simulink model "gm_sampleModel71194_pp_7_1_sub"  (R2023b)
settings: Solver=VariableStepAuto  StartTime=0.0  StopTime=10.0  RelTol=1e-3
libraries: simulink x45, hdlsllib x1, hdlmdlgenlib x1
(part 2 of 2)

== system gm_sampleModel71194_pp_7_1_sub/Subsystem/cfblk214 ==
  emi_180 : Inport  OutDataTypeStr=boolean  PortDimensions=1  SampleTime=1
  Action Port : Inport  Port=2  OutDataTypeStr=boolean  SampleTime=1
  cfblk214 : DataTypeConversion  OutDataTypeStr=uint8  SampleTime=1  SaturateOnIntegerOverflow=off  RndMeth=Floor
  cfblk214_out1bypassMux : MultiPortSwitch  DataPortOrder=Zero-based contiguous  Inputs=2  zeroidx=on  OutDataTypeStr=uint8  SampleTime=1  SaturateOnIntegerOverflow=off  InputSameDT=off
  emi_181_bypass : UnitDelay  InitialCondition="fi(0,0,8,0,\"hex\",\"00\")"  SampleTime=1
  emi_181 : Outport  SampleTime=1  InitialOutput=0
  wires:
  Action Port/1 -> cfblk214_out1bypassMux/1
  emi_180/1 -> cfblk214/1
  cfblk214/1 -> cfblk214_out1bypassMux/3
  cfblk214_out1bypassMux/1 -> emi_181_bypass/1, emi_181/1
  emi_181_bypass/1 -> cfblk214_out1bypassMux/2

== system gm_sampleModel71194_pp_7_1_sub/Subsystem/cfblk216 ==
  emi_188 : Inport  OutDataTypeStr=uint8  PortDimensions=1  SampleTime=1
  Action Port : Inport  Port=2  OutDataTypeStr=boolean  SampleTime=1
  cfblk216 : DataTypeConversion  OutDataTypeStr=fixdt(0,8,0)
  cfblk216_out1bypassMux : MultiPortSwitch  DataPortOrder=Zero-based contiguous  Inputs=2  zeroidx=on  OutDataTypeStr=uint8  SampleTime=1  SaturateOnIntegerOverflow=off  InputSameDT=off
  emi_189_bypass : UnitDelay  InitialCondition="fi(0,0,8,0,\"hex\",\"00\")"  SampleTime=1
  emi_189 : Outport  SampleTime=1  InitialOutput=0
  wires:
  Action Port/1 -> cfblk216_out1bypassMux/1
  emi_188/1 -> cfblk216/1
  cfblk216/1 -> cfblk216_out1bypassMux/3
  cfblk216_out1bypassMux/1 -> emi_189_bypass/1, emi_189/1
  emi_189_bypass/1 -> cfblk216_out1bypassMux/2

== system gm_sampleModel71194_pp_7_1_sub/Subsystem/cfblk217 ==
  emi_196 : Inport  OutDataTypeStr=fixdt(0, 16, 7)  PortDimensions=1  SampleTime=1
  Action Port : Inport  Port=2  OutDataTypeStr=boolean  SampleTime=1
  cfblk217 : DataTypeConversion  OutDataTypeStr=uint8  SampleTime=1  SaturateOnIntegerOverflow=off  RndMeth=Floor
  cfblk217_out1bypassMux : MultiPortSwitch  DataPortOrder=Zero-based contiguous  Inputs=2  zeroidx=on  OutDataTypeStr=uint8  SampleTime=1  SaturateOnIntegerOverflow=off  InputSameDT=off
  emi_197_bypass : UnitDelay  InitialCondition="fi(0,0,8,0,\"hex\",\"00\")"  SampleTime=1
  emi_197 : Outport  SampleTime=1  InitialOutput=0
  wires:
  Action Port/1 -> cfblk217_out1bypassMux/1
  emi_196/1 -> cfblk217/1
  cfblk217/1 -> cfblk217_out1bypassMux/3
  cfblk217_out1bypassMux/1 -> emi_197_bypass/1, emi_197/1
  emi_197_bypass/1 -> cfblk217_out1bypassMux/2

== system gm_sampleModel71194_pp_7_1_sub/Subsystem/cfblk220 ==
  emi_230 : Inport  OutDataTypeStr=uint8  PortDimensions=1  SampleTime=1
  Action Port : Inport  Port=2  OutDataTypeStr=boolean  SampleTime=1
  cfblk220 : DataTypeConversion  OutDataTypeStr=fixdt(0,8,0)
  cfblk220_out1bypassMux : MultiPortSwitch  DataPortOrder=Zero-based contiguous  Inputs=2  zeroidx=on  OutDataTypeStr=uint8  SampleTime=1  SaturateOnIntegerOverflow=off  InputSameDT=off
  emi_231_bypass : UnitDelay  InitialCondition="fi(0,0,8,0,\"hex\",\"00\")"  SampleTime=1
  emi_231 : Outport  SampleTime=1  InitialOutput=0
  wires:
  Action Port/1 -> cfblk220_out1bypassMux/1
  emi_230/1 -> cfblk220/1
  cfblk220/1 -> cfblk220_out1bypassMux/3
  cfblk220_out1bypassMux/1 -> emi_231_bypass/1, emi_231/1
  emi_231_bypass/1 -> cfblk220_out1bypassMux/2

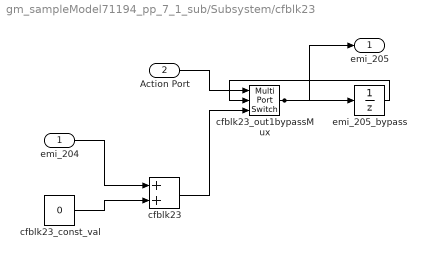
== system gm_sampleModel71194_pp_7_1_sub/Subsystem/cfblk23 ==
  emi_204 : Inport  OutDataTypeStr=uint8  PortDimensions=1  SampleTime=1
  Action Port : Inport  Port=2  OutDataTypeStr=boolean  SampleTime=1
  cfblk23 : Sum  OutDataTypeStr=uint8  AccumDataTypeStr=uint8  RndMeth=Nearest  SampleTime=1
  cfblk23_const_val : Constant  Value=0  VectorParams1D=off  OutDataTypeStr=uint8  SampleTime=1
  cfblk23_out1bypassMux : MultiPortSwitch  DataPortOrder=Zero-based contiguous  Inputs=2  zeroidx=on  OutDataTypeStr=uint8  SampleTime=1  SaturateOnIntegerOverflow=off  InputSameDT=off
  emi_205_bypass : UnitDelay  InitialCondition="fi(0,0,8,0,\"hex\",\"00\")"  SampleTime=1
  emi_205 : Outport  SampleTime=1  InitialOutput=0
  wires:
  Action Port/1 -> cfblk23_out1bypassMux/1
  emi_204/1 -> cfblk23/1
  cfblk23/1 -> cfblk23_out1bypassMux/3
  cfblk23_out1bypassMux/1 -> emi_205_bypass/1, emi_205/1
  emi_205_bypass/1 -> cfblk23_out1bypassMux/2
  cfblk23_const_val/1 -> cfblk23/2

== system gm_sampleModel71194_pp_7_1_sub/Subsystem/cfblk27 ==
  emi_164 : Inport  OutDataTypeStr=uint8  PortDimensions=1  SampleTime=1
  Action Port : Inport  Port=2  OutDataTypeStr=boolean  SampleTime=1
  cfblk27 : Abs  SampleTime=1  OutDataTypeStr=uint8  SaturateOnIntegerOverflow=off
  cfblk27_out1bypassMux : MultiPortSwitch  DataPortOrder=Zero-based contiguous  Inputs=2  zeroidx=on  OutDataTypeStr=uint8  SampleTime=1  SaturateOnIntegerOverflow=off  InputSameDT=off
  emi_165_bypass : UnitDelay  InitialCondition="fi(0,0,8,0,\"hex\",\"00\")"  SampleTime=1
  emi_165 : Outport  SampleTime=1  InitialOutput=0
  wires:
  Action Port/1 -> cfblk27_out1bypassMux/1
  emi_164/1 -> cfblk27/1
  cfblk27/1 -> cfblk27_out1bypassMux/3
  cfblk27_out1bypassMux/1 -> emi_165_bypass/1, emi_165/1
  emi_165_bypass/1 -> cfblk27_out1bypassMux/2

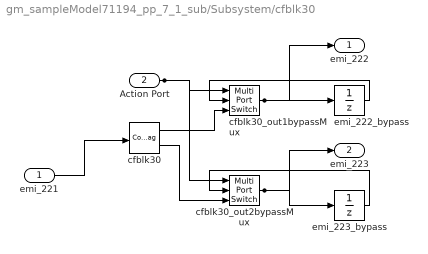
== system gm_sampleModel71194_pp_7_1_sub/Subsystem/cfblk30 ==
  emi_221 : Inport  OutDataTypeStr=uint8  PortDimensions=1  SampleTime=1
  Action Port : Inport  Port=2  OutDataTypeStr=boolean  SampleTime=1
  cfblk30 : ComplexToRealImag  SampleTime=1
  cfblk30_out1bypassMux : MultiPortSwitch  DataPortOrder=Zero-based contiguous  Inputs=2  zeroidx=on  OutDataTypeStr=uint8  SampleTime=1  SaturateOnIntegerOverflow=off  InputSameDT=off
  cfblk30_out2bypassMux : MultiPortSwitch  DataPortOrder=Zero-based contiguous  Inputs=2  zeroidx=on  OutDataTypeStr=uint8  SampleTime=1  SaturateOnIntegerOverflow=off  InputSameDT=off
  emi_222_bypass : UnitDelay  InitialCondition="fi(0,0,8,0,\"hex\",\"00\")"  SampleTime=1
  emi_223_bypass : UnitDelay  InitialCondition="fi(0,0,8,0,\"hex\",\"00\")"  SampleTime=1
  emi_222 : Outport  SampleTime=1  InitialOutput=0
  emi_223 : Outport  Port=2  SampleTime=1  InitialOutput=0
  wires:
  Action Port/1 -> cfblk30_out2bypassMux/1, cfblk30_out1bypassMux/1
  emi_221/1 -> cfblk30/1
  cfblk30/1 -> cfblk30_out1bypassMux/3
  cfblk30/2 -> cfblk30_out2bypassMux/3
  cfblk30_out1bypassMux/1 -> emi_222_bypass/1, emi_222/1
  emi_222_bypass/1 -> cfblk30_out1bypassMux/2
  cfblk30_out2bypassMux/1 -> emi_223_bypass/1, emi_223/1
  emi_223_bypass/1 -> cfblk30_out2bypassMux/2

== system gm_sampleModel71194_pp_7_1_sub/Subsystem/cfblk31_inst ==
  in1 : Inport  OutDataTypeStr=uint8  SampleTime=1
  in2 : Inport  Port=2  OutDataTypeStr=uint8  SampleTime=1
  mul_cfblk31_dotp_mulcomp : Product  Inputs=**  OutDataTypeStr=uint8  SampleTime=1
  out1 : Outport  OutDataTypeStr=uint8  SampleTime=1
  wires:
  in1/1 -> mul_cfblk31_dotp_mulcomp/1
  in2/1 -> mul_cfblk31_dotp_mulcomp/2
  mul_cfblk31_dotp_mulcomp/1 -> out1/1

== system gm_sampleModel71194_pp_7_1_sub/Subsystem/cfblk37 ==
  emi_238 : Inport  OutDataTypeStr=uint8  PortDimensions=1  SampleTime=1
  Action Port : Inport  Port=2  OutDataTypeStr=boolean  SampleTime=1
  cfblk37 : MinMax
  cfblk37_out1bypassMux : MultiPortSwitch  DataPortOrder=Zero-based contiguous  Inputs=2  zeroidx=on  OutDataTypeStr=uint8  SampleTime=1  SaturateOnIntegerOverflow=off  InputSameDT=off
  emi_239_bypass : UnitDelay  InitialCondition="fi(0,0,8,0,\"hex\",\"00\")"  SampleTime=1
  emi_239 : Outport  SampleTime=1  InitialOutput=0
  wires:
  Action Port/1 -> cfblk37_out1bypassMux/1
  emi_238/1 -> cfblk37/1
  cfblk37/1 -> cfblk37_out1bypassMux/3
  cfblk37_out1bypassMux/1 -> emi_239_bypass/1, emi_239/1
  emi_239_bypass/1 -> cfblk37_out1bypassMux/2

== system gm_sampleModel71194_pp_7_1_sub/Subsystem/cfblk38 ==
  u : Inport  OutDataTypeStr=uint8  SampleTime=1
  FixPt Constant : Constant  DisableCoverage=on  OutDataTypeStr=Inherit: Inherit via back propagation  SampleTime=-1
  FixPt Data Type Duplicate : DataTypeDuplicate  DisableCoverage=on  NumInputPorts=3
  FixPt Sum1 : Sum  OutDataTypeStr=Inherit: Inherit via back propagation  InputSameDT=on  LockScale=on
  y : Outport  SampleTime=1
  wires:
  u/1 -> FixPt Sum1/1, FixPt Data Type Duplicate/2
  FixPt Constant/1 -> FixPt Sum1/2, FixPt Data Type Duplicate/3
  FixPt Sum1/1 -> FixPt Data Type Duplicate/1, y/1

== system gm_sampleModel71194_pp_7_1_sub/Subsystem/cfblk39 ==
  emi_246 : Inport  OutDataTypeStr=uint8  PortDimensions=1  SampleTime=1
  Action Port : Inport  Port=2  OutDataTypeStr=boolean  SampleTime=1
  cfblk39 : Subsystem  mask(Real World Value Increment){}
      mask help: Simulink:masks:RealWorldValueIncrement_MD
      mask Display: disp('V++')
  cfblk39_out1bypassMux : MultiPortSwitch  DataPortOrder=Zero-based contiguous  Inputs=2  zeroidx=on  OutDataTypeStr=uint8  SampleTime=1  SaturateOnIntegerOverflow=off  InputSameDT=off
  emi_247_bypass : UnitDelay  InitialCondition="fi(0,0,8,0,\"hex\",\"00\")"  SampleTime=1
  emi_247 : Outport  SampleTime=1  InitialOutput=0
  wires:
  Action Port/1 -> cfblk39_out1bypassMux/1
  emi_246/1 -> cfblk39/1(u)
  cfblk39/1(y) -> cfblk39_out1bypassMux/3
  cfblk39_out1bypassMux/1 -> emi_247_bypass/1, emi_247/1
  emi_247_bypass/1 -> cfblk39_out1bypassMux/2

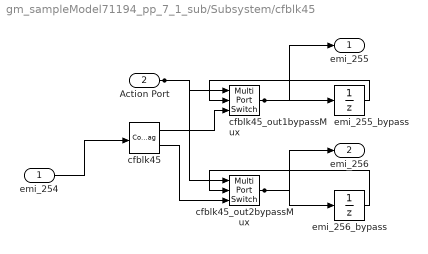
== system gm_sampleModel71194_pp_7_1_sub/Subsystem/cfblk45 ==
  emi_254 : Inport  OutDataTypeStr=uint8  PortDimensions=1  SampleTime=1
  Action Port : Inport  Port=2  OutDataTypeStr=boolean  SampleTime=1
  cfblk45 : ComplexToRealImag  SampleTime=1
  cfblk45_out1bypassMux : MultiPortSwitch  DataPortOrder=Zero-based contiguous  Inputs=2  zeroidx=on  OutDataTypeStr=uint8  SampleTime=1  SaturateOnIntegerOverflow=off  InputSameDT=off
  cfblk45_out2bypassMux : MultiPortSwitch  DataPortOrder=Zero-based contiguous  Inputs=2  zeroidx=on  OutDataTypeStr=uint8  SampleTime=1  SaturateOnIntegerOverflow=off  InputSameDT=off
  emi_255_bypass : UnitDelay  InitialCondition="fi(0,0,8,0,\"hex\",\"00\")"  SampleTime=1
  emi_256_bypass : UnitDelay  InitialCondition="fi(0,0,8,0,\"hex\",\"00\")"  SampleTime=1
  emi_255 : Outport  SampleTime=1  InitialOutput=0
  emi_256 : Outport  Port=2  SampleTime=1  InitialOutput=0
  wires:
  Action Port/1 -> cfblk45_out2bypassMux/1, cfblk45_out1bypassMux/1
  emi_254/1 -> cfblk45/1
  cfblk45/1 -> cfblk45_out1bypassMux/3
  cfblk45/2 -> cfblk45_out2bypassMux/3
  cfblk45_out1bypassMux/1 -> emi_255_bypass/1, emi_255/1
  emi_255_bypass/1 -> cfblk45_out1bypassMux/2
  cfblk45_out2bypassMux/1 -> emi_256_bypass/1, emi_256/1
  emi_256_bypass/1 -> cfblk45_out2bypassMux/2

== system gm_sampleModel71194_pp_7_1_sub/Subsystem/cfblk46 ==
  emi_263 : Inport  OutDataTypeStr=uint8  PortDimensions=1  SampleTime=1
  Action Port : Inport  Port=2  OutDataTypeStr=boolean  SampleTime=1
  cfblk46 : Sum  Inputs=+
  cfblk46_out1bypassMux : MultiPortSwitch  DataPortOrder=Zero-based contiguous  Inputs=2  zeroidx=on  OutDataTypeStr=uint8  SampleTime=1  SaturateOnIntegerOverflow=off  InputSameDT=off
  emi_264_bypass : UnitDelay  InitialCondition="fi(0,0,8,0,\"hex\",\"00\")"  SampleTime=1
  emi_264 : Outport  SampleTime=1  InitialOutput=0
  wires:
  Action Port/1 -> cfblk46_out1bypassMux/1
  emi_263/1 -> cfblk46/1
  cfblk46/1 -> cfblk46_out1bypassMux/3
  cfblk46_out1bypassMux/1 -> emi_264_bypass/1, emi_264/1
  emi_264_bypass/1 -> cfblk46_out1bypassMux/2

== system gm_sampleModel71194_pp_7_1_sub/Subsystem/cfblk50 ==
  emi_271 : Inport  OutDataTypeStr=uint8  PortDimensions=1  SampleTime=1
  Action Port : Inport  Port=2  OutDataTypeStr=boolean  SampleTime=1
  cfblk50 : Sum  Inputs=+
  cfblk50_out1bypassMux : MultiPortSwitch  DataPortOrder=Zero-based contiguous  Inputs=2  zeroidx=on  OutDataTypeStr=uint8  SampleTime=1  SaturateOnIntegerOverflow=off  InputSameDT=off
  emi_272_bypass : UnitDelay  InitialCondition="fi(0,0,8,0,\"hex\",\"00\")"  SampleTime=1
  emi_272 : Outport  SampleTime=1  InitialOutput=0
  wires:
  Action Port/1 -> cfblk50_out1bypassMux/1
  emi_271/1 -> cfblk50/1
  cfblk50/1 -> cfblk50_out1bypassMux/3
  cfblk50_out1bypassMux/1 -> emi_272_bypass/1, emi_272/1
  emi_272_bypass/1 -> cfblk50_out1bypassMux/2

== system gm_sampleModel71194_pp_7_1_sub/Subsystem/cfblk52 ==
  u : Inport  OutDataTypeStr=uint8  SampleTime=1
  FixPt Constant : Constant  DisableCoverage=on  OutDataTypeStr=Inherit: Inherit via back propagation  SampleTime=-1
  FixPt Data Type Duplicate : DataTypeDuplicate  DisableCoverage=on  NumInputPorts=3
  FixPt Sum1 : Sum  OutDataTypeStr=Inherit: Inherit via back propagation  InputSameDT=on  LockScale=on
  y : Outport  SampleTime=1
  wires:
  u/1 -> FixPt Sum1/1, FixPt Data Type Duplicate/2
  FixPt Constant/1 -> FixPt Sum1/2, FixPt Data Type Duplicate/3
  FixPt Sum1/1 -> FixPt Data Type Duplicate/1, y/1

== system gm_sampleModel71194_pp_7_1_sub/Subsystem/cfblk54 ==
  emi_279 : Inport  OutDataTypeStr=uint8  PortDimensions=1  SampleTime=1
  Action Port : Inport  Port=2  OutDataTypeStr=boolean  SampleTime=1
  cfblk54 : MinMax
  cfblk54_out1bypassMux : MultiPortSwitch  DataPortOrder=Zero-based contiguous  Inputs=2  zeroidx=on  OutDataTypeStr=uint8  SampleTime=1  SaturateOnIntegerOverflow=off  InputSameDT=off
  emi_280_bypass : UnitDelay  InitialCondition="fi(0,0,8,0,\"hex\",\"00\")"  SampleTime=1
  emi_280 : Outport  SampleTime=1  InitialOutput=0
  wires:
  Action Port/1 -> cfblk54_out1bypassMux/1
  emi_279/1 -> cfblk54/1
  cfblk54/1 -> cfblk54_out1bypassMux/3
  cfblk54_out1bypassMux/1 -> emi_280_bypass/1, emi_280/1
  emi_280_bypass/1 -> cfblk54_out1bypassMux/2

== system gm_sampleModel71194_pp_7_1_sub/Subsystem/cfblk55 ==
  u : Inport  OutDataTypeStr=uint8  SampleTime=1
  FixPt Constant : Constant  DisableCoverage=on  OutDataTypeStr=Inherit: Inherit via back propagation  SampleTime=-1
  FixPt Data Type Duplicate : DataTypeDuplicate  DisableCoverage=on  NumInputPorts=3
  FixPt Sum1 : Sum  OutDataTypeStr=Inherit: Inherit via back propagation  InputSameDT=on  LockScale=on
  y : Outport  SampleTime=1
  wires:
  u/1 -> FixPt Sum1/1, FixPt Data Type Duplicate/2
  FixPt Constant/1 -> FixPt Sum1/2, FixPt Data Type Duplicate/3
  FixPt Sum1/1 -> FixPt Data Type Duplicate/1, y/1

== system gm_sampleModel71194_pp_7_1_sub/Subsystem/cfblk6 ==
  emi_287 : Inport  OutDataTypeStr=boolean  PortDimensions=1  SampleTime=1
  Action Port : Inport  Port=2  OutDataTypeStr=boolean  SampleTime=1
  cfblk6 : simulink/Logic and Bit Operations/Bitwise Operator  logicop=AND  UseBitMask=on  BitMask="fi(0,0,1,0,\"hex\",\"1\")"  BitMaskRealWorld=Real World Value
  cfblk6_out1bypassMux : MultiPortSwitch  DataPortOrder=Zero-based contiguous  Inputs=2  zeroidx=on  SampleTime=1  SaturateOnIntegerOverflow=off  InputSameDT=off
  emi_288_bypass : UnitDelay  SampleTime=1
  emi_288 : Outport  SampleTime=1  InitialOutput=0
  wires:
  Action Port/1 -> cfblk6_out1bypassMux/1
  emi_287/1 -> cfblk6/1
  cfblk6/1 -> cfblk6_out1bypassMux/3
  cfblk6_out1bypassMux/1 -> emi_288_bypass/1, emi_288/1
  emi_288_bypass/1 -> cfblk6_out1bypassMux/2

== system gm_sampleModel71194_pp_7_1_sub/Subsystem/cfblk60 ==
  u : Inport  OutDataTypeStr=uint8  SampleTime=1
  FixPt Constant : Constant  DisableCoverage=on  OutDataTypeStr=Inherit: Inherit via back propagation  SampleTime=-1
  FixPt Data Type Duplicate : DataTypeDuplicate  DisableCoverage=on  NumInputPorts=3
  FixPt Sum1 : Sum  OutDataTypeStr=Inherit: Inherit via back propagation  InputSameDT=on  LockScale=on
  y : Outport  SampleTime=1
  wires:
  u/1 -> FixPt Sum1/1, FixPt Data Type Duplicate/2
  FixPt Constant/1 -> FixPt Sum1/2, FixPt Data Type Duplicate/3
  FixPt Sum1/1 -> FixPt Data Type Duplicate/1, y/1

== system gm_sampleModel71194_pp_7_1_sub/Subsystem/cfblk63 ==
  emi_295 : Inport  OutDataTypeStr=uint8  PortDimensions=1  SampleTime=1
  Action Port : Inport  Port=2  OutDataTypeStr=boolean  SampleTime=1
  cfblk63 : Subsystem  mask(Real World Value Increment){}
      mask help: Simulink:masks:RealWorldValueIncrement_MD
      mask Display: disp('V++')
  cfblk63_out1bypassMux : MultiPortSwitch  DataPortOrder=Zero-based contiguous  Inputs=2  zeroidx=on  OutDataTypeStr=uint8  SampleTime=1  SaturateOnIntegerOverflow=off  InputSameDT=off
  emi_296_bypass : UnitDelay  InitialCondition="fi(0,0,8,0,\"hex\",\"00\")"  SampleTime=1
  emi_296 : Outport  SampleTime=1  InitialOutput=0
  wires:
  Action Port/1 -> cfblk63_out1bypassMux/1
  emi_295/1 -> cfblk63/1(u)
  cfblk63/1(y) -> cfblk63_out1bypassMux/3
  cfblk63_out1bypassMux/1 -> emi_296_bypass/1, emi_296/1
  emi_296_bypass/1 -> cfblk63_out1bypassMux/2

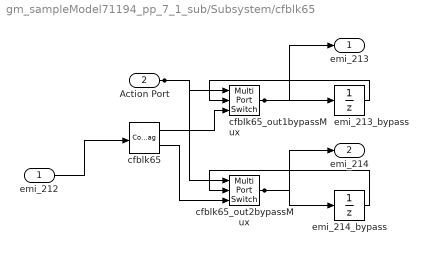
== system gm_sampleModel71194_pp_7_1_sub/Subsystem/cfblk65 ==
  emi_212 : Inport  OutDataTypeStr=uint8  PortDimensions=1  SampleTime=1
  Action Port : Inport  Port=2  OutDataTypeStr=boolean  SampleTime=1
  cfblk65 : ComplexToRealImag  SampleTime=1
  cfblk65_out1bypassMux : MultiPortSwitch  DataPortOrder=Zero-based contiguous  Inputs=2  zeroidx=on  OutDataTypeStr=uint8  SampleTime=1  SaturateOnIntegerOverflow=off  InputSameDT=off
  cfblk65_out2bypassMux : MultiPortSwitch  DataPortOrder=Zero-based contiguous  Inputs=2  zeroidx=on  OutDataTypeStr=uint8  SampleTime=1  SaturateOnIntegerOverflow=off  InputSameDT=off
  emi_213_bypass : UnitDelay  InitialCondition="fi(0,0,8,0,\"hex\",\"00\")"  SampleTime=1
  emi_214_bypass : UnitDelay  InitialCondition="fi(0,0,8,0,\"hex\",\"00\")"  SampleTime=1
  emi_213 : Outport  SampleTime=1  InitialOutput=0
  emi_214 : Outport  Port=2  SampleTime=1  InitialOutput=0
  wires:
  Action Port/1 -> cfblk65_out2bypassMux/1, cfblk65_out1bypassMux/1
  emi_212/1 -> cfblk65/1
  cfblk65/1 -> cfblk65_out1bypassMux/3
  cfblk65/2 -> cfblk65_out2bypassMux/3
  cfblk65_out1bypassMux/1 -> emi_213_bypass/1, emi_213/1
  emi_213_bypass/1 -> cfblk65_out1bypassMux/2
  cfblk65_out2bypassMux/1 -> emi_214_bypass/1, emi_214/1
  emi_214_bypass/1 -> cfblk65_out2bypassMux/2

== system gm_sampleModel71194_pp_7_1_sub/Subsystem/cfblk67 ==
  emi_303 : Inport  OutDataTypeStr=uint8  PortDimensions=1  SampleTime=1
  Action Port : Inport  Port=2  OutDataTypeStr=boolean  SampleTime=1
  cfblk67 : Subsystem  mask(Real World Value Increment){}
      mask help: Simulink:masks:RealWorldValueIncrement_MD
      mask Display: disp('V++')
  cfblk67_out1bypassMux : MultiPortSwitch  DataPortOrder=Zero-based contiguous  Inputs=2  zeroidx=on  OutDataTypeStr=uint8  SampleTime=1  SaturateOnIntegerOverflow=off  InputSameDT=off
  emi_304_bypass : UnitDelay  InitialCondition="fi(0,0,8,0,\"hex\",\"00\")"  SampleTime=1
  emi_304 : Outport  SampleTime=1  InitialOutput=0
  wires:
  Action Port/1 -> cfblk67_out1bypassMux/1
  emi_303/1 -> cfblk67/1(u)
  cfblk67/1(y) -> cfblk67_out1bypassMux/3
  cfblk67_out1bypassMux/1 -> emi_304_bypass/1, emi_304/1
  emi_304_bypass/1 -> cfblk67_out1bypassMux/2

== system gm_sampleModel71194_pp_7_1_sub/Subsystem/cfblk7 ==
  u : Inport  OutDataTypeStr=uint8  SampleTime=1
  Compare : RelationalOperator  Operator=<=  OutDataTypeStr=fixdt(0, 8)
  Constant : Constant  DisableCoverage=on  Value=0  OutDataTypeStr=Inherit: Inherit via back propagation  SampleTime=-1  PreserveConstantTs=on
  y : Outport  SampleTime=1
  wires:
  u/1 -> Compare/1
  Compare/1 -> y/1
  Constant/1 -> Compare/2

== system gm_sampleModel71194_pp_7_1_sub/Subsystem/cfblk75 ==
  u : Inport  OutDataTypeStr=uint8  SampleTime=1
  FixPt Constant : Constant  DisableCoverage=on  OutDataTypeStr=Inherit: Inherit via back propagation  SampleTime=-1
  FixPt Data Type Duplicate : DataTypeDuplicate  DisableCoverage=on  NumInputPorts=3
  FixPt Sum1 : Sum  OutDataTypeStr=Inherit: Inherit via back propagation  InputSameDT=on  LockScale=on
  y : Outport  SampleTime=1
  wires:
  u/1 -> FixPt Sum1/1, FixPt Data Type Duplicate/2
  FixPt Constant/1 -> FixPt Sum1/2, FixPt Data Type Duplicate/3
  FixPt Sum1/1 -> FixPt Data Type Duplicate/1, y/1

== system gm_sampleModel71194_pp_7_1_sub/Subsystem/cfblk87_inst ==
  in1 : Inport  OutDataTypeStr=uint8  SampleTime=1
  in2 : Inport  Port=2  OutDataTypeStr=uint8  SampleTime=1
  mul_cfblk87_dotp_mulcomp : Product  Inputs=**  OutDataTypeStr=uint8  SampleTime=1
  out1 : Outport  OutDataTypeStr=uint8  SampleTime=1
  wires:
  in1/1 -> mul_cfblk87_dotp_mulcomp/1
  in2/1 -> mul_cfblk87_dotp_mulcomp/2
  mul_cfblk87_dotp_mulcomp/1 -> out1/1

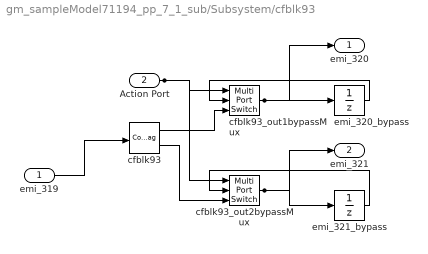
== system gm_sampleModel71194_pp_7_1_sub/Subsystem/cfblk93 ==
  emi_319 : Inport  OutDataTypeStr=uint8  PortDimensions=1  SampleTime=1
  Action Port : Inport  Port=2  OutDataTypeStr=boolean  SampleTime=1
  cfblk93 : ComplexToRealImag  SampleTime=1
  cfblk93_out1bypassMux : MultiPortSwitch  DataPortOrder=Zero-based contiguous  Inputs=2  zeroidx=on  OutDataTypeStr=uint8  SampleTime=1  SaturateOnIntegerOverflow=off  InputSameDT=off
  cfblk93_out2bypassMux : MultiPortSwitch  DataPortOrder=Zero-based contiguous  Inputs=2  zeroidx=on  OutDataTypeStr=uint8  SampleTime=1  SaturateOnIntegerOverflow=off  InputSameDT=off
  emi_320_bypass : UnitDelay  InitialCondition="fi(0,0,8,0,\"hex\",\"00\")"  SampleTime=1
  emi_321_bypass : UnitDelay  InitialCondition="fi(0,0,8,0,\"hex\",\"00\")"  SampleTime=1
  emi_320 : Outport  SampleTime=1  InitialOutput=0
  emi_321 : Outport  Port=2  SampleTime=1  InitialOutput=0
  wires:
  Action Port/1 -> cfblk93_out2bypassMux/1, cfblk93_out1bypassMux/1
  emi_319/1 -> cfblk93/1
  cfblk93/1 -> cfblk93_out1bypassMux/3
  cfblk93/2 -> cfblk93_out2bypassMux/3
  cfblk93_out1bypassMux/1 -> emi_320_bypass/1, emi_320/1
  emi_320_bypass/1 -> cfblk93_out1bypassMux/2
  cfblk93_out2bypassMux/1 -> emi_321_bypass/1, emi_321/1
  emi_321_bypass/1 -> cfblk93_out2bypassMux/2

== system gm_sampleModel71194_pp_7_1_sub/Subsystem/cfblk95 ==
  emi_311 : Inport  OutDataTypeStr=uint8  PortDimensions=1  SampleTime=1
  Action Port : Inport  Port=2  OutDataTypeStr=boolean  SampleTime=1
  cfblk95 : Signum  SampleTime=1
  cfblk95_out1bypassMux : MultiPortSwitch  DataPortOrder=Zero-based contiguous  Inputs=2  zeroidx=on  OutDataTypeStr=uint8  SampleTime=1  SaturateOnIntegerOverflow=off  InputSameDT=off
  emi_312_bypass : UnitDelay  InitialCondition="fi(0,0,8,0,\"hex\",\"00\")"  SampleTime=1
  emi_312 : Outport  SampleTime=1  InitialOutput=0
  wires:
  Action Port/1 -> cfblk95_out1bypassMux/1
  emi_311/1 -> cfblk95/1
  cfblk95/1 -> cfblk95_out1bypassMux/3
  cfblk95_out1bypassMux/1 -> emi_312_bypass/1, emi_312/1
  emi_312_bypass/1 -> cfblk95_out1bypassMux/2

== system gm_sampleModel71194_pp_7_1_sub/Subsystem/cfblk103/cfblk103 ==
  u : Inport  OutDataTypeStr=uint8  SampleTime=1
  FixPt Constant : Constant  DisableCoverage=on  OutDataTypeStr=Inherit: Inherit via back propagation  SampleTime=-1
  FixPt Data Type Duplicate : DataTypeDuplicate  DisableCoverage=on  NumInputPorts=3
  FixPt Sum1 : Sum  OutDataTypeStr=Inherit: Inherit via back propagation  InputSameDT=on  LockScale=on
  y : Outport  SampleTime=1  InitialOutput=0
  wires:
  u/1 -> FixPt Sum1/1, FixPt Data Type Duplicate/2
  FixPt Constant/1 -> FixPt Sum1/2, FixPt Data Type Duplicate/3
  FixPt Sum1/1 -> FixPt Data Type Duplicate/1, y/1

== system gm_sampleModel71194_pp_7_1_sub/Subsystem/cfblk11/cfblk11 ==
  note: Edge
  note: U(k)
  U : Inport  OutDataTypeStr=uint8  SampleTime=1
  Action Port_out2 : Inport  Port=2  OutDataTypeStr=boolean  SampleTime=1
  Delay Input1 : Subsystem
      settings: MinAlgLoopOccurrences=on
  FixPt Relational Operator : RelationalOperator  Operator=<  OutDataTypeStr=fixdt(0,8,0)  SampleTime=1  InputSameDT=off
  Y : Outport  SampleTime=1  InitialOutput=0
  wires:
  U/1 -> FixPt Relational Operator/1, Delay Input1/1(in0)
  Delay Input1/1(out0) -> FixPt Relational Operator/2
  FixPt Relational Operator/1 -> Y/1
  Action Port_out2/1 -> Delay Input1/Enable

== system gm_sampleModel71194_pp_7_1_sub/Subsystem/cfblk130/cfblk130 ==
  u : Inport  OutDataTypeStr=uint8  SampleTime=1
  FixPt Constant : Constant  DisableCoverage=on  OutDataTypeStr=Inherit: Inherit via back propagation  SampleTime=-1
  FixPt Data Type Duplicate : DataTypeDuplicate  DisableCoverage=on  NumInputPorts=3
  FixPt Sum1 : Sum  OutDataTypeStr=Inherit: Inherit via back propagation  InputSameDT=on  LockScale=on
  y : Outport  SampleTime=1  InitialOutput=0
  wires:
  u/1 -> FixPt Sum1/1, FixPt Data Type Duplicate/2
  FixPt Constant/1 -> FixPt Sum1/2, FixPt Data Type Duplicate/3
  FixPt Sum1/1 -> FixPt Data Type Duplicate/1, y/1

== system gm_sampleModel71194_pp_7_1_sub/Subsystem/cfblk14/Nonpositive ==
  u : Inport  OutDataTypeStr=uint8  SampleTime=1
  Compare : RelationalOperator  Operator=<=  OutDataTypeStr=boolean  ZeroCross=off
  Constant : Constant  DisableCoverage=on  Value=0  OutDataTypeStr=Inherit: Inherit via back propagation  SampleTime=-1  PreserveConstantTs=on
  y : Outport  SampleTime=1
  wires:
  u/1 -> Compare/1
  Compare/1 -> y/1
  Constant/1 -> Compare/2

== system gm_sampleModel71194_pp_7_1_sub/Subsystem/cfblk153/cfblk153 ==
  u : Inport  OutDataTypeStr=uint8  SampleTime=1
  FixPt Constant : Constant  DisableCoverage=on  OutDataTypeStr=Inherit: Inherit via back propagation  SampleTime=-1
  FixPt Data Type Duplicate : DataTypeDuplicate  DisableCoverage=on  NumInputPorts=3
  FixPt Sum1 : Sum  OutDataTypeStr=Inherit: Inherit via back propagation  InputSameDT=on  LockScale=on
  y : Outport  SampleTime=1  InitialOutput=0
  wires:
  u/1 -> FixPt Sum1/1, FixPt Data Type Duplicate/2
  FixPt Constant/1 -> FixPt Sum1/2, FixPt Data Type Duplicate/3
  FixPt Sum1/1 -> FixPt Data Type Duplicate/1, y/1

== system gm_sampleModel71194_pp_7_1_sub/Subsystem/cfblk174/cfblk174 ==
  in0 : Inport  OutDataTypeStr=uint8  SampleTime=1
  Action Port_out2 : EnablePort  OutDataTypeStr=boolean
  cfblk174 : Delay  DelayLength=double(2)  InitialCondition=0
  out0 : Outport  OutDataTypeStr=uint8  SampleTime=1  InitialOutput=0
  wires:
  cfblk174/1 -> out0/1
  in0/1 -> cfblk174/1

== system gm_sampleModel71194_pp_7_1_sub/Subsystem/cfblk2/cfblk2 ==
  u : Inport  OutDataTypeStr=uint8  SampleTime=1
  Compare : RelationalOperator  Operator=<=  OutDataTypeStr=fixdt(0, 8)
  Constant : Constant  DisableCoverage=on  Value=const  OutDataTypeStr=Inherit: Inherit via back propagation  SampleTime=-1
  y : Outport  SampleTime=1  InitialOutput=0
  wires:
  u/1 -> Compare/1
  Compare/1 -> y/1
  Constant/1 -> Compare/2

== system gm_sampleModel71194_pp_7_1_sub/Subsystem/cfblk39/cfblk39 ==
  u : Inport  OutDataTypeStr=uint8  SampleTime=1
  FixPt Constant : Constant  DisableCoverage=on  OutDataTypeStr=Inherit: Inherit via back propagation  SampleTime=-1
  FixPt Data Type Duplicate : DataTypeDuplicate  DisableCoverage=on  NumInputPorts=3
  FixPt Sum1 : Sum  OutDataTypeStr=Inherit: Inherit via back propagation  InputSameDT=on  LockScale=on
  y : Outport  SampleTime=1  InitialOutput=0
  wires:
  u/1 -> FixPt Sum1/1, FixPt Data Type Duplicate/2
  FixPt Constant/1 -> FixPt Sum1/2, FixPt Data Type Duplicate/3
  FixPt Sum1/1 -> FixPt Data Type Duplicate/1, y/1

== system gm_sampleModel71194_pp_7_1_sub/Subsystem/cfblk63/cfblk63 ==
  u : Inport  OutDataTypeStr=uint8  SampleTime=1
  FixPt Constant : Constant  DisableCoverage=on  OutDataTypeStr=Inherit: Inherit via back propagation  SampleTime=-1
  FixPt Data Type Duplicate : DataTypeDuplicate  DisableCoverage=on  NumInputPorts=3
  FixPt Sum1 : Sum  OutDataTypeStr=Inherit: Inherit via back propagation  InputSameDT=on  LockScale=on
  y : Outport  SampleTime=1  InitialOutput=0
  wires:
  u/1 -> FixPt Sum1/1, FixPt Data Type Duplicate/2
  FixPt Constant/1 -> FixPt Sum1/2, FixPt Data Type Duplicate/3
  FixPt Sum1/1 -> FixPt Data Type Duplicate/1, y/1

== system gm_sampleModel71194_pp_7_1_sub/Subsystem/cfblk67/cfblk67 ==
  u : Inport  OutDataTypeStr=uint8  SampleTime=1
  FixPt Constant : Constant  DisableCoverage=on  OutDataTypeStr=Inherit: Inherit via back propagation  SampleTime=-1
  FixPt Data Type Duplicate : DataTypeDuplicate  DisableCoverage=on  NumInputPorts=3
  FixPt Sum1 : Sum  OutDataTypeStr=Inherit: Inherit via back propagation  InputSameDT=on  LockScale=on
  y : Outport  SampleTime=1  InitialOutput=0
  wires:
  u/1 -> FixPt Sum1/1, FixPt Data Type Duplicate/2
  FixPt Constant/1 -> FixPt Sum1/2, FixPt Data Type Duplicate/3
  FixPt Sum1/1 -> FixPt Data Type Duplicate/1, y/1

== system gm_sampleModel71194_pp_7_1_sub/Subsystem/cfblk11/cfblk11/Delay Input1 ==
  in0 : Inport  OutDataTypeStr=uint8  SampleTime=1
  Action Port_out2 : EnablePort  OutDataTypeStr=boolean
  Delay Input1 : Delay  DelayLength=double(1)  InitialCondition=0
  out0 : Outport  OutDataTypeStr=uint8  SampleTime=1  InitialOutput=0
  wires:
  Delay Input1/1 -> out0/1
  in0/1 -> Delay Input1/1
